simulink model "Stabilization_PI"  (Simulink 7.8)
settings: Solver=ode4  StartTime=Tstart  StopTime=Tfinal  FixedStep=Ts  RelTol=1e-3
values from neighbouring files (symbols this model uses):
  Ki_omega = r_omega*W_omega^2 / (Km*Wm^2)    [Automatic_Control.m]
  Km = num_motor(3) / den_motor(3)    [Automatic_Control.m]    (also in Gimbal_Motor_Modeling.m = (num_m(3))/den_m(3))
  Kp_omega = ( 2*Z_omega*W_omega*r_omega + W_omega^2 - Wm^2) / (Km*Wm^2)    [Automatic_Control.m]
  Ts = 0.005    [Automatic_Control.m]
  Wm = den_motor(3)^0.5    [Automatic_Control.m]    (also in Gimbal_Motor_Modeling.m = (den_m(3))^0.5)
  Zm = den_motor(2) / 2 / Wm    [Automatic_Control.m]    (also in Gimbal_Motor_Modeling.m = (den_m(2)) / 2 / Wm)
undefined symbols (not defined in the file or in its folder): z_den, z_num
settings Model: Creator=mechatronics  LastModifiedBy=mechatronics
settings SolverCC: AutoInsertRateTranBlk=on

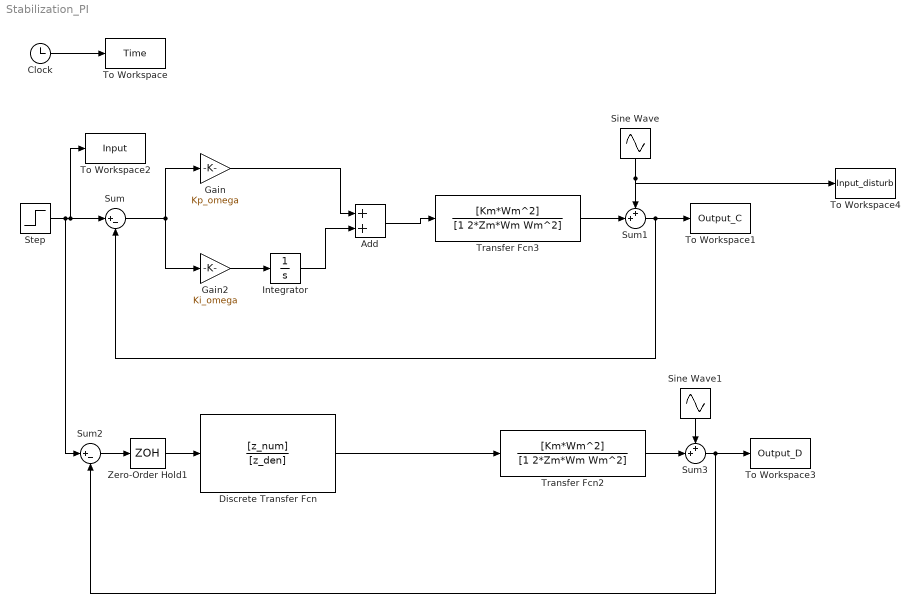
== system Stabilization_PI ==
  Add : Sum
  Clock : Clock
  Discrete Transfer Fcn : DiscreteTransferFcn  Numerator=[z_num]  Denominator=[z_den]  SampleTime=-1
  Gain : Gain  Gain=Kp_omega
  Gain2 : Gain  Gain=Ki_omega
  Integrator : Integrator
  Sine Wave : Sin  Amplitude=0  Frequency=0.5*2*pi  SampleTime=0
  Sine Wave1 : Sin  Amplitude=0  Frequency=0.5*2*pi  SampleTime=0
  Step : Step  Time=0  SampleTime=0
  Sum : Sum  Inputs=|+-
  Sum1 : Sum  Inputs=++|
  Sum2 : Sum  Inputs=|+-
  Sum3 : Sum  Inputs=++|
  To Workspace : ToWorkspace  VariableName=Time  SampleTime=-1  SaveFormat=Array
  To Workspace1 : ToWorkspace  VariableName=Output_C  SampleTime=-1  SaveFormat=Array
  To Workspace2 : ToWorkspace  VariableName=Input  SampleTime=-1  SaveFormat=Array
  To Workspace3 : ToWorkspace  VariableName=Output_D  SampleTime=-1  SaveFormat=Array
  To Workspace4 : ToWorkspace  VariableName=Input_disturb  SampleTime=-1  SaveFormat=Array
  Transfer Fcn2 : TransferFcn  Numerator=[Km*Wm^2]  Denominator=[1 2*Zm*Wm Wm^2]
  Transfer Fcn3 : TransferFcn  Numerator=[Km*Wm^2]  Denominator=[1 2*Zm*Wm Wm^2]
  Zero-Order Hold1 : ZeroOrderHold  SampleTime=Ts
  wires:
  Clock/1 -> To Workspace/1
  Gain2/1 -> Integrator/1
  Sum/1 -> Gain/1, Gain2/1
  Gain/1 -> Add/1
  Integrator/1 -> Add/2
  Step/1 -> Sum/1, To Workspace2/1, Sum2/1
  Add/1 -> Transfer Fcn3/1
  Transfer Fcn3/1 -> Sum1/2
  Sine Wave/1 -> Sum1/1, To Workspace4/1
  Sum1/1 -> To Workspace1/1, Sum/2
  Transfer Fcn2/1 -> Sum3/2
  Sine Wave1/1 -> Sum3/1
  Sum3/1 -> Sum2/2, To Workspace3/1
  Sum2/1 -> Zero-Order Hold1/1
  Zero-Order Hold1/1 -> Discrete Transfer Fcn/1
  Discrete Transfer Fcn/1 -> Transfer Fcn2/1
